simulink model "AAI_proof_of_concept"  (R2020a)
settings: Solver=FixedStepAuto  StartTime=0.0  StopTime=10.0  FixedStep=1e-3  RelTol=1e-3  EnableMultiTasking=on
settings Model: ExtModeTrigDuration=5  Creator=Ethan  LastModifiedBy=Ethan
settings OptimizationCC: EnhancedBackFolding=on  PassReuseOutputArgsAs=Individual arguments  ZeroExternalMemoryAtStartup=off  ZeroInternalMemoryAtStartup=off  MaxStackSize=64  OptimizeBlockOrder=speed  DifferentSizesBufferReuse=on  OptimizationCustomize=off  EfficientTunableParamExpr=on
settings DebuggingCC: ParameterTunabilityLossMsg=error
settings HardwareCC: ProdBitPerPointer=32  ProdBitPerSizeT=32  ProdBitPerPtrDiffT=32  ProdLargestAtomicInteger=Long  ProdLargestAtomicFloat=Double  ProdWordSize=32  ProdHWDeviceType=ARM Compatible->ARM Cortex
settings SFSimCC: MATLABDynamicMemAlloc=off
settings RTWCC: SystemTargetFile=ert.tlc  HardwareBoard=NXP FRDM-K64F  TemplateMakefile=ert_default_tmf  Toolchain=GNU Tools for ARM Embedded Processors
settings CodeAppCC: ForceParamTrailComments=on  IgnoreCustomStorageClasses=off  OperatorAnnotations=on  SimulinkDataObjDesc=on  SFDataObjDesc=on  InsertBlockDesc=on

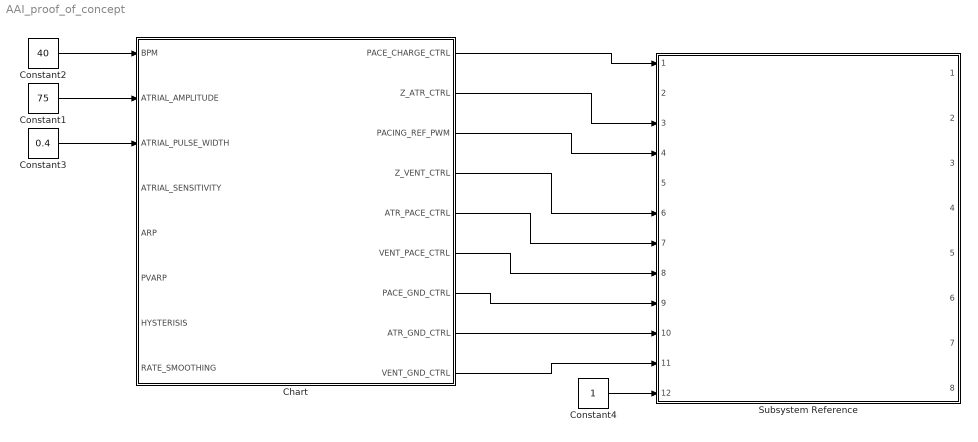
== system AAI_proof_of_concept ==
  Chart : Stateflow chart  TreatAsAtomicUnit=on
      settings: PortSchema="{\"entries\":[{\"content\":{\"sides\":[{\"content\":{\"connectorIds\":[\"In1\",\"In2\",\"In3\",\"In4\",\"In5\",\"In6\",\"In7\",\"In8\"]},\"type\":\"ConnectorPlacement.EquallySpacedRectSide\",\"uuid\":\"b678de6f-9e61-4024-a0aa-5bf6d03f3d0b\"},{\"content\":{\"connectorIds\":[\"Out3\",\"Out8\",\"Out5\",\"Out9\",\"Out2\",\"Out7\",\"Out4\",\"Out1\",\"Out6\"],\"side\":\"RIGHT\"},\"type\":\"ConnectorPlacement.EquallySpacedRectSide\",\"uuid\":\"4cd0faad-dd9d-4a56-81c5-44f7dd4bee31\"},{\"content\":{\"connectorIds\":[],\"side\":\"TOP\"},\"type\":\"ConnectorPlacement.EquallySpacedRectSide\",\"uuid\":\"a9bc4227-6f84-42c8-b827-a378e14304fe\"}]},\"type\":\"ConnectorPlacement.EquallySpacedConnector\",\"uuid\":\"ee3b07ee-2423-4f21-89d4-53b7a563517d\"}],\"packageUris\":[\"http://schema.mathworks.com/mf0/Connector/19700101\"],\"version\":\"1.0\"}"
  Constant1 : Constant  Value=75
  Constant2 : Constant  Value=40
  Constant3 : Constant  Value=0.4
  Constant4 : Constant
  Subsystem Reference : Subsystem  ReferencedSubsystem=k64f_subsystem
  wires:
  Chart/9(Z_VENT_CTRL) -> Subsystem Reference/6
  Chart/5(PACING_REF_PWM) -> Subsystem Reference/4
  Chart/7(VENT_PACE_CTRL) -> Subsystem Reference/8
  Chart/6(VENT_GND_CTRL) -> Subsystem Reference/11
  Constant2/1 -> Chart/1(BPM)
  Chart/2(ATR_PACE_CTRL) -> Subsystem Reference/7
  Chart/1(ATR_GND_CTRL) -> Subsystem Reference/10
  Chart/8(Z_ATR_CTRL) -> Subsystem Reference/3
  Chart/3(PACE_CHARGE_CTRL) -> Subsystem Reference/1
  Chart/4(PACE_GND_CTRL) -> Subsystem Reference/9
  Constant1/1 -> Chart/2(ATRIAL_AMPLITUDE)
  Constant3/1 -> Chart/3(ATRIAL_PULSE_WIDTH)
  Constant4/1 -> Subsystem Reference/12

== stateflow chart AAI_proof_of_concept/Chart ==
  state PULSE_ATR
    entry:
    PACE_CHARGE_CTRL = 0;
    PACE_GND_CTRL = 1;
    VENT_GND_CTRL = 0;
    VENT_PACE_CTRL = 0;
    Z_ATR_CTRL = 0;
    Z_VENT_CTRL = 0;
    ATR_GND_CTRL = 0;
    ATR_PACE_CTRL = 1;
  state CHARGE
    entry:
    ATR_PACE_CTRL = 0;
    VENT_PACE_CTRL = 0;
    PACING_REF_PWM = ATRIAL_AMPLITUDE;
    PACE_CHARGE_CTRL = 1;
  state DISCHARGE
    entry:
    PACE_GND_CTRL = 1;
    VENT_PACE_CTRL = 0;
    Z_ATR_CTRL = 0;
    Z_VENT_CTRL = 0;
    ATR_PACE_CTRL = 0;
    ATR_GND_CTRL = 0;
    VENT_GND_CTRL = 1;
  (default) -> CHARGE
  CHARGE -> PULSE_ATR : after(60/BPM,sec)
  DISCHARGE -> CHARGE
  PULSE_ATR -> DISCHARGE : after(ATRIAL_PULSE_WIDTH, msec)
  data: ATR_GND_CTRL output; ATR_PACE_CTRL output; PACE_CHARGE_CTRL output; PACE_GND_CTRL output; PACING_REF_PWM output; VENT_GND_CTRL output; VENT_PACE_CTRL output; Z_ATR_CTRL output; Z_VENT_CTRL output; BPM input; ATRIAL_AMPLITUDE input; ATRIAL_PULSE_WIDTH input; ATRIAL_SENSITIVITY input; ARP input; PVARP input; HYSTERISIS input; RATE_SMOOTHING input
